simulink model "atv2"  (R2022a)
settings: Solver=VariableStepAuto  StartTime=0.0  StopTime=50  RelTol=1e-3
settings Model: Creator=a2103303  LastModifiedBy=a2103303

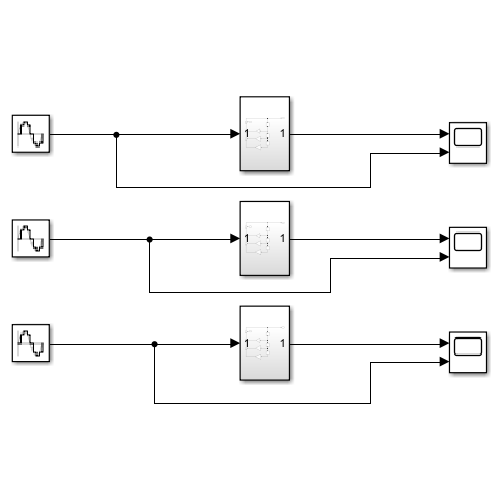
[thumbnail: Simulink's stored preview of the top-level diagram]
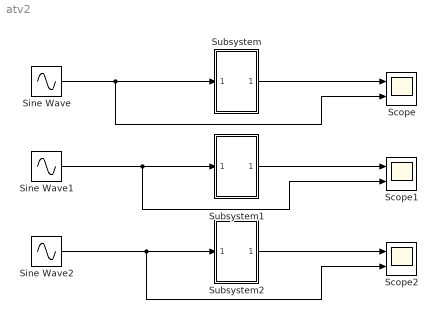
== system atv2 ==
  Scope : Scope  NumInputPorts=2
  Scope1 : Scope  NumInputPorts=2
  Scope2 : Scope  NumInputPorts=2
  Sine Wave : Sin  Frequency=3.14/4  SampleTime=1
  Sine Wave1 : Sin  Frequency=3.14/2  SampleTime=1
  Sine Wave2 : Sin  Frequency=(3*3.14)/4  SampleTime=1
  Subsystem : Subsystem
  Subsystem1 : Subsystem
  Subsystem2 : Subsystem
  wires:
  Subsystem/1(Out1) -> Scope/1
  Sine Wave1/1 -> Scope1/2, Subsystem1/1(In1)
  Sine Wave/1 -> Scope/2, Subsystem/1(In1)
  Sine Wave2/1 -> Scope2/2, Subsystem2/1(In1)
  Subsystem1/1(Out1) -> Scope1/1
  Subsystem2/1(Out1) -> Scope2/1

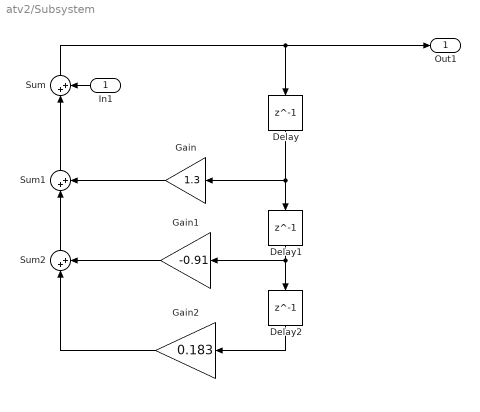
== system atv2/Subsystem ==
  In1 : Inport
  Delay : Delay  DelayLength=1  InitialCondition=0
  Delay1 : Delay  DelayLength=1  InitialCondition=0
  Delay2 : Delay  DelayLength=1  InitialCondition=0
  Gain : Gain  Gain=1.3
  Gain1 : Gain  Gain=-0.91
  Gain2 : Gain  Gain=0.183
  Sum : Sum  Inputs=|++
  Sum1 : Sum  Inputs=|++
  Sum2 : Sum  Inputs=|++
  Out1 : Outport
  wires:
  Gain1/1 -> Sum2/2
  Sum1/1 -> Sum/1
  Delay1/1 -> Delay2/1, Gain1/1
  Delay/1 -> Delay1/1, Gain/1
  Gain2/1 -> Sum2/1
  Sum2/1 -> Sum1/1
  Sum/1 -> Out1/1, Delay/1
  In1/1 -> Sum/2
  Gain/1 -> Sum1/2
  Delay2/1 -> Gain2/1

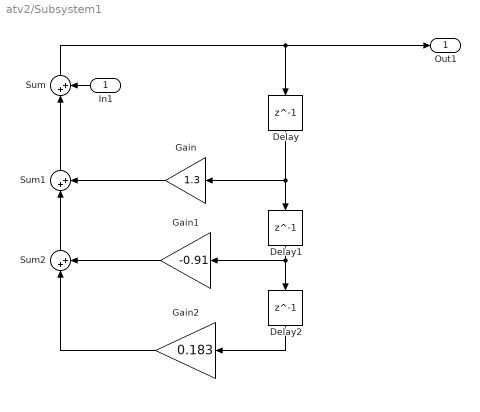
== system atv2/Subsystem1 ==
  In1 : Inport
  Delay : Delay  DelayLength=1  InitialCondition=0
  Delay1 : Delay  DelayLength=1  InitialCondition=0
  Delay2 : Delay  DelayLength=1  InitialCondition=0
  Gain : Gain  Gain=1.3
  Gain1 : Gain  Gain=-0.91
  Gain2 : Gain  Gain=0.183
  Sum : Sum  Inputs=|++
  Sum1 : Sum  Inputs=|++
  Sum2 : Sum  Inputs=|++
  Out1 : Outport
  wires:
  Gain1/1 -> Sum2/2
  Sum1/1 -> Sum/1
  Delay1/1 -> Delay2/1, Gain1/1
  Delay/1 -> Delay1/1, Gain/1
  Gain2/1 -> Sum2/1
  Sum2/1 -> Sum1/1
  Sum/1 -> Out1/1, Delay/1
  In1/1 -> Sum/2
  Gain/1 -> Sum1/2
  Delay2/1 -> Gain2/1

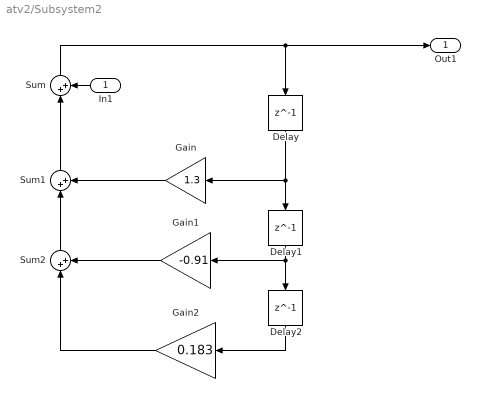
== system atv2/Subsystem2 ==
  In1 : Inport
  Delay : Delay  DelayLength=1  InitialCondition=0
  Delay1 : Delay  DelayLength=1  InitialCondition=0
  Delay2 : Delay  DelayLength=1  InitialCondition=0
  Gain : Gain  Gain=1.3
  Gain1 : Gain  Gain=-0.91
  Gain2 : Gain  Gain=0.183
  Sum : Sum  Inputs=|++
  Sum1 : Sum  Inputs=|++
  Sum2 : Sum  Inputs=|++
  Out1 : Outport
  wires:
  Gain1/1 -> Sum2/2
  Sum1/1 -> Sum/1
  Delay1/1 -> Delay2/1, Gain1/1
  Delay/1 -> Delay1/1, Gain/1
  Gain2/1 -> Sum2/1
  Sum2/1 -> Sum1/1
  Sum/1 -> Out1/1, Delay/1
  In1/1 -> Sum/2
  Gain/1 -> Sum1/2
  Delay2/1 -> Gain2/1
